simulink model "discrete_model"  (R2022b)
settings: Solver=FixedStepAuto  StartTime=0.0  StopTime=.5  FixedStep=0.0001  RelTol=1e-3
values from neighbouring files (symbols this model uses):
  A = [0 1 0; a21 0 a23; a31 0 a33]    [ex5.m]
  a21 = 1/(2*m)*x30^2*FemP1/FemP2^2*exp(-x10/FemP2)    [ex5.m]
  a23 = -1/(m)*x30*FemP1/FemP2*exp(-x10/FemP2)    [ex5.m]
  a31 = 1/f1*exp(x10/f2)*(ki*u10+ci-x30)    [ex5.m]
  a33 = -f2/f1*exp(x10/f2)    [ex5.m]
  B = [0 0; 0 g; b31 0]    [ex5.m]
  b31 = ki*f2/f1*exp(x10/f2)    [ex5.m]
  C = [1 0 0]    [ex5.m]
  g = 9.81    [ex5.m]
  Kx = -acker(A, B(:,1), -sKx)    [ex5.m]
  u0 = -(a31*x1+a33*x3)/b31    [ex5.m]
  u10 = 1/ki*(x30-ci)    [ex5.m]
  x1 = .003    (= 0.003)    [ex5.m]
  x2 = 0    [ex5.m]
  x3 = -(a21*x1+g)/a23    [ex5.m]
  xd = d-bd    (= 0.0192)    [ex5.m]
settings Model: Creator=MPatr  LastModifiedBy=MPatr

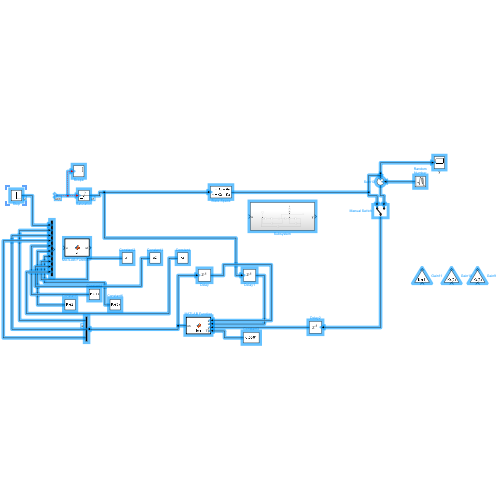
[thumbnail: Simulink's stored preview of the top-level diagram]
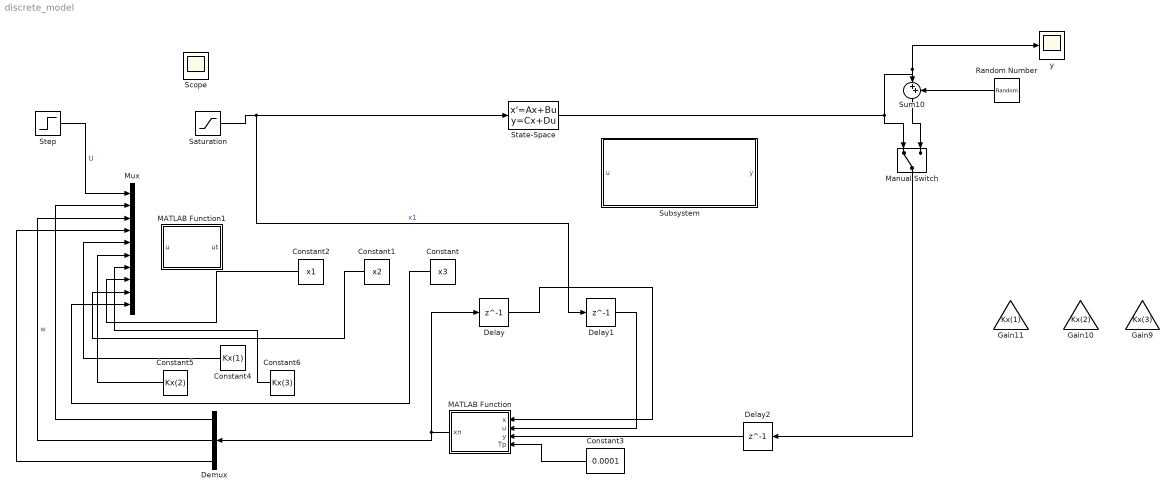
== system discrete_model ==
  Constant : Constant  Value=x3
  Constant1 : Constant  Value=x2
  Constant2 : Constant  Value=x1
  Constant3 : Constant  Value=0.0001
  Constant4 : Constant  Value=Kx(1)
  Constant5 : Constant  Value=Kx(2)
  Constant6 : Constant  Value=Kx(3)
  Delay : Delay  DelayLength=1
  Delay1 : Delay  DelayLength=1
  Delay2 : Delay  DelayLength=1
  Demux : Demux  Outputs=3
  Gain10 : Gain  Gain=Kx(2)
  Gain11 : Gain  Gain=Kx(1)
  Gain9 : Gain  Gain=Kx(3)
  MATLAB Function : MATLAB Function  TreatAsAtomicUnit=on
  MATLAB Function1 : MATLAB Function  TreatAsAtomicUnit=on
  Manual Switch : ManualSwitch
  Mux : Mux  Inputs=10
  Random Number : RandomNumber  Variance=.0000001
  Saturation : Saturate  UpperLimit=1  LowerLimit=0
  Scope : Scope
  State-Space : StateSpace  A=A  B=B  C=C  D=[0 0]  InitialCondition=0
  Step : Step  Time=0  Before=u10  After=u0  SampleTime=0
  Subsystem : Subsystem
  Sum10 : Sum  Inputs=|++
  y : Scope
  wires:
  Saturation/1 -> State-Space/1, Delay1/1  "x1"
  Manual Switch/1 -> Delay2/1
  Random Number/1 -> Sum10/2
  Sum10/1 -> Manual Switch/2
  State-Space/1 -> y/1, Sum10/1, Manual Switch/1
  Step/1 -> Mux/1  "U"
  ? -> Saturation/1, Scope/1  "uz(t)"
  MATLAB Function/1(xn) -> Delay/1, Demux/1
  Delay/1 -> MATLAB Function/1(x)
  Delay1/1 -> MATLAB Function/2(u)
  Delay2/1 -> MATLAB Function/3(y)
  Constant3/1 -> MATLAB Function/4(Tp)
  Demux/3 -> Mux/4
  Demux/2 -> Mux/3  "w"
  Demux/1 -> Mux/2
  Constant4/1 -> Mux/5
  Constant5/1 -> Mux/6
  Constant6/1 -> Mux/7
  Constant2/1 -> Mux/8
  Constant1/1 -> Mux/9
  Constant/1 -> Mux/10

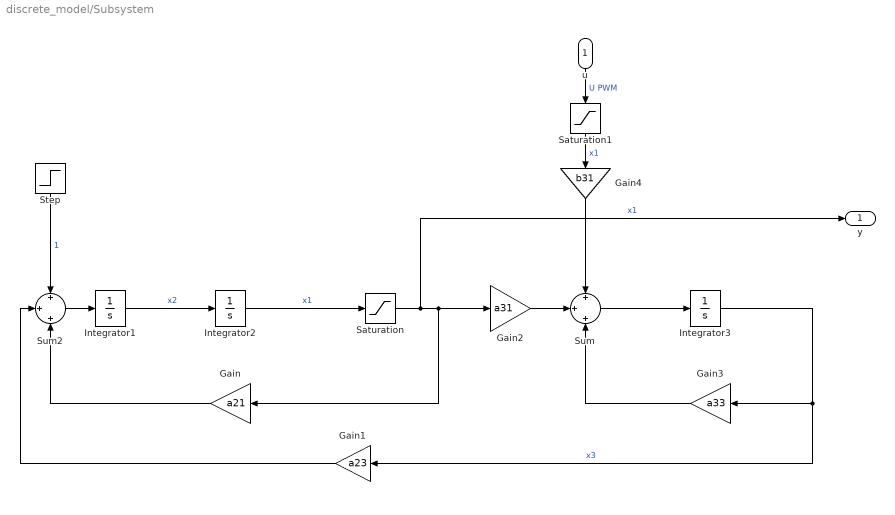
== system discrete_model/Subsystem ==
  u : Inport
  Gain : Gain  Gain=a21
  Gain1 : Gain  Gain=a23
  Gain2 : Gain  Gain=a31
  Gain3 : Gain  Gain=a33
  Gain4 : Gain  Gain=b31
  Integrator1 : Integrator
  Integrator2 : Integrator  InitialCondition=xd
  Integrator3 : Integrator
  Saturation : Saturate  UpperLimit=xd  LowerLimit=0
  Saturation1 : Saturate  UpperLimit=1  LowerLimit=0
  Step : Step  Time=0  After=g  SampleTime=0
  Sum : Sum  Inputs=+|+|+
  Sum2 : Sum  Inputs=+|+|+
  y : Outport
  wires:
  Step/1 -> Sum2/1  "1"
  Integrator1/1 -> Integrator2/1  "x2"
  Gain1/1 -> Sum2/2
  u/1 -> Saturation1/1  "U PWM"
  Saturation/1 -> y/1, Gain2/1, Gain/1  "x1"
  Integrator3/1 -> Gain3/1, Gain1/1  "x3"
  Gain/1 -> Sum2/3
  Gain2/1 -> Sum/2
  Gain3/1 -> Sum/3
  Sum2/1 -> Integrator1/1
  Sum/1 -> Integrator3/1
  Integrator2/1 -> Saturation/1  "x1"
  Gain4/1 -> Sum/1
  Saturation1/1 -> Gain4/1  "x1"

== matlab function discrete_model/MATLAB Function1 ==
  data: u input; ut output
function ut  = fcn(u)
yr = u(1);
x = [u(2); u(3); u(4)];
k = [u(5), u(6), u(7)];
xr = [u(8); u(9); u(10)];

utt = yr + k*(x-xr);

ut = [utt; 1];

== matlab function discrete_model/MATLAB Function ==
  data: x input; u input; y input; Tp input; xn output
function xn  = fcn(x, u, y, Tp)

m = .00575;
g = 9.81;
FemP1 = .017521;
FemP2 = .0058231;
f1 = .00014142;
f2 = .0045626;
ki = 2.5165;
ci = .0243 * sign(4-2);
d = .0792;
bd = .06;
xd = d-bd;
x10 = .008;
x20 = 0;
x30 = .75;
u10 = 1/ki*(x30-ci);
% 0.2883767137

a21 = 1/(2*m)*x30^2*FemP1/FemP2^2*exp(-x10/FemP2); 
a23 = -1/(m)*x30*FemP1/FemP2*exp(-x10/FemP2); 
a31 = 1/f1*exp(x10/f2)*(ki*u10+ci-x30); 
a33 = -f2/f1*exp(x10/f2);
b31 = ki*f2/f1*exp(x10/f2);
A = [0 1 0; a21 0 a23; a31 0 a33];
B = [0 0; 0 g; b31 0];
C = [1 0 0];
D = 0;

% sLo = 200*ones(1,3)
Lo = [-44.6; 60.0; 65.0];

xnt = (eye(3)+A*Tp)*x + B*Tp*u + Lo*Tp*(y-C*x)

xn = xnt(:, 1)
